simulink model "ISReferenceApplication"  (R2018a)
settings: Solver=FixedStepAuto  StartTime=0  StopTime=Tend  FixedStep=0.001  RelTol=5e-3
model workspace (MAT data in the model file):
  A_mu = 10
  B_reff = 8.386
  Cz = 7766.25
  DCT_Param.Transmission.Ratios = [3.78 2.18 1.43 1.03 0.935 0.84]
  DCT_Param.Transmission.Shaft_Inertia_Odd = 0.0023
  DCT_Param.Transmission.Shaft_Inertia_Even = 0.0009
  DCT_Param.Transmission.Shaft_Inertia_Output = 0.008
  DCT_Param.Transmission.Gear_Inertia = 0.001
  DCT_Param.Transmission.Gear_Efficiency = 0.94
  DCT_Param.Transmission.Gear_Ang_Vel_Thr = 0.01
  DCT_Param.Transmission.Shaft_Velocity_Odd = 0
  DCT_Param.Transmission.Shaft_Velocity_Even = 0
  DCT_Param.Transmission.Shaft_Velocity_Output = 0
  DCT_Param.Transmission.Gear_Initial_Velocity = 0
  DCT_Param.Transmission.Abstract.Compliance = 100000
  DCT_Param.Transmission.Abstract.Damping = 10000
  DCT_Param.Transmission.Abstract.Ratio_Time_Const = 0.05
  DCT_Param.Transmission.Abstract.Shift_Gear_Delay = 25
  DCT_Param.Clutch.Torque_Radius = 130
  DCT_Param.Clutch.Num_Friction_Surfaces = 4
  DCT_Param.Clutch.Engagement_Piston_Area = 0.001
  DCT_Param.Clutch.Kinetic_Friction_Coeff = 0.3
  DCT_Param.Clutch.Static_Friction_Coeff = 0.31
  DCT_Param.Clutch.Derating_Factor = 1
  DCT_Param.Clutch.Clutch_Velocity_Tolerance = 0.001
  DCT_Param.Clutch.Threshold_Pressure = 1
  DCT_Param.Clutch.Drag_Torque_Coeff = 0
  DCT_Param.Dog_Clutch.Max_Torque = 1000
  DCT_Param.Dog_Clutch.Teeth_Mean_Radius = 50
  DCT_Param.Dog_Clutch.Tooth_Height = 10
  DCT_Param.Dog_Clutch.Ring_Hub_Clearance = 3
  DCT_Param.Dog_Clutch.Ring_Stop_Stiffness = 1000000
  DCT_Param.Dog_Clutch.Ring_Stop_Damping = 1000
  DCT_Param.Dog_Clutch.Shift_Linkage_Damping = 100
  DCT_Param.Dog_Clutch.Max_Engage_Velocity = 1000000
  DCT_Param.Dog_Clutch.Tooth_Engage_Overlap = 3
  DCT_Param.Vehicle.Mass = 1600
  DCT_Param.Vehicle.Wheels_Per_Axle = 2
  DCT_Param.Vehicle.Distance_CG_FrontAxle = 1.7
  DCT_Param.Vehicle.Distance_CG_RearAxle = 2
  DCT_Param.Vehicle.Distance_CG_Ground = 0.5
  DCT_Param.Vehicle.Frontal_Area = 3
  DCT_Param.Vehicle.Aero_Drag_Coeff = 0.4
  DCT_Param.Vehicle.Initial_Velocity = 0
  DCT_Param.Vehicle.Final_Drive_Ratio = 3.7
  DCT_Param.Vehicle.Final_Drive_Efficiency = 0.86
  DCT_Param.Vehicle.Final_Drive_Vel_Thresh = 0.01
  DCT_Param.Vehicle.Side_Shaft_Inertia = 0.01
  DCT_Param.Vehicle.Side_Shaft_Initial_Velocity = 0
  DCT_Param.Vehicle.Tire.Radius = 0.312
  DCT_Param.Vehicle.Tire.Inertia = 0.5
  DCT_Param.Vehicle.Tire.Initial_Velocity = 0
  DCT_Param.Vehicle.Tire.Slip_Vel_Thresh = 0.1
  DCT_Param.Vehicle.Tire.Nominal_Vertical_Load = 4000
  DCT_Param.Vehicle.Tire.C_Coeff = 1.685
  DCT_Param.Vehicle.Tire.D_Coeff = [1.21 -0.037]
  DCT_Param.Vehicle.Tire.E_Coeff = [0.344 0.095 -0.02 0]
  DCT_Param.Vehicle.Tire.BCD_Coeff = [21.51 -0.163 0.245]
  DCT_Param.Vehicle.Tire.H_Coeff = [-0.002 0.002]
  DCT_Param.Vehicle.Tire.V_Coeff = [0 0]
  DCT_Param.ICE.Max_Power = 100000
  DCT_Param.ICE.Speed_At_Max_Power = 5500
  DCT_Param.ICE.Max_Speed = 7000
  DCT_Param.ICE.Stall_Speed = 200
  DCT_Param.ICE.Shaft_Inertia = 0.2
  DCT_Param.ICE.Initial_Velocity = 800
  DCT_Param.ICE.Idle_Ref_Spd = 800
  DCT_Param.ICE.Engine_Time_Constant = 0.2
  DCT_Param.ICE.Initial_Normalized_Throttle = 0
  DCT_Param.ICE.Speed_Threshold = 20
  DCT_Param.ICE.FC.Speed_Vector = [0 368.421052632 736.842105263 1105.26315789 1473.68421053 1842.10526316 2210.52631579 2578.94736842 2947.36842105 3315.78947368 3684.21052632 4052.63157895 4421.05263158 4789.47368421 5157.89473684 5526.31578947 5894.73684211 6263.15789474 6631.57894737 7000]
  DCT_Param.ICE.FC.Torque_Vector = [0 10.5263157895 21.0526315789 31.5789473684 42.1052631579 52.6315789474 63.1578947368 73.6842105263 84.2105263158 94.7368421053 105.263157895 115.789473684 126.315789474 136.842105263 147.368421053 157.894736842 168.421052632 178.947368421 189.473684211 200]
  DCT_Param.ICE.FC.Consumption_Table = [0.262945178015 0.225304787522 0.201465019624 0.191425874321 0.195187351614 0.212749451502 0.244112173984 0.289275519063 0.348239486736 0.421004077004 0.507569289868 0.607935125326 ... (400 elements, 20x20)]
  DCT_Param.Shift_Map_Example.Pedal_Positions = [0.1 0.4 0.5 0.9]
  DCT_Param.Shift_Map_Example.Upshift_Speeds = [11  20  26  34.5  43; 14  26  35  44.5  55; 17  31  42  52.5  65; 21  39  52  66.5  80]
  DCT_Param.Shift_Map_Example.Downshift_Speeds = [8.9  17  23.6  32.4  40.8; 11.5  22.7  32  41.6  52.2; 14  27  38.1  50  62; 18  33  48  62.6  76.2]
  DCT_Param.Shift_Map_ORIG.Pedal_Positions = [0.1 0.4 0.5 0.9]
  DCT_Param.Shift_Map_ORIG.Upshift_Speeds = [11.5  23.5  35.5  45.5  55.5; 14.5  26.5  38.5  48.5  58.5; 17.5  29.5  41.5  51.5  61.5; 20.5  32.5  44.5  54.5  64.5]
  DCT_Param.Shift_Map_ORIG.Downshift_Speeds = [8.5  20.5  32.5  42.5  52.5; 11.5  23.5  35.5  45.5  55.5; 14.5  26.5  38.5  48.5  58.5; 17.5  29.5  41.5  51.5  61.5]
  DCT_Param.Shift_Map_OPT.Pedal_Positions = [0.1 0.4 0.5 0.9]
  DCT_Param.Shift_Map_OPT.Upshift_Speeds = [17.8469  29.8469  35.8159  41.2981  46.3004; 19.2469  33.9778  43.9778  53.9778  63.9778; 24.5469  41.9778  62.1778  78.5778  106.9778; 27.5469  59.3778  99.0445  109.0445  119.0445]
  DCT_Param.Shift_Map_OPT.Downshift_Speeds = [14.8469  26.8469  32.8159  38.2981  43.3004; 16.2469  30.9778  40.9778  50.9778  60.9778; 21.5469  38.9778  59.1778  75.5778  103.9778; 24.5469  56.3778  96.0445  106.0445  116.0445]
  DCT_Param.Shift_Map.Pedal_Positions = [0.1 0.4 0.5 0.9]
  DCT_Param.Shift_Map.Upshift_Speeds = [11.5  23.5  35.5  45.5  55.5; 14.5  26.5  38.5  48.5  58.5; 17.5  29.5  41.5  51.5  61.5; 20.5  32.5  44.5  54.5  64.5]
  DCT_Param.Shift_Map.Downshift_Speeds = [8.5  20.5  32.5  42.5  52.5; 11.5  23.5  35.5  45.5  55.5; 14.5  26.5  38.5  48.5  58.5; 17.5  29.5  41.5  51.5  61.5]
  DCT_Param.Control.Clutch.Min_Lock_Pressure = 2000000
  DCT_Param.Control.Clutch.Max_Lock_Pressure = 5000000
  DCT_Param.Control.Clutch.Max_Unlock_Pressure = 500000
  DCT_Param.Control.Engine_Start_RPM = 800
  DCT_Param.Control.Engine_Stop_RPM = 790
  DCT_Param.Control.Mode_Logic_TS = 0.1
  DCT_Param.Control.ICE.Kp = 0.02
  DCT_Param.Control.ICE.Ki = 0.01
  DCT_Param.Control.Gen.Kp = 10
  DCT_Param.Control.Gen.Ki = 3
  DCT_Param.Control.Mot.Kp = 500
  DCT_Param.Control.Mot.Ki = 300
  DCT_Param.Control.Veh_Spd.Kp = 0.02
  DCT_Param.Control.Veh_Spd.Ki = 0.04
  DCT_Param.Driver.Kp = 400
  DCT_Param.Driver.Ki = 0.001
  DCT_Param.Driver.Pedal_Filter_Const = 0.01
  DCT_Param.Dog_Clutches.Pulse_Delay = 50
  DCT_Param.Dog_Clutches.Pulse_Length = 20
  DCT_Param.Animation.Teeth_Ratios = [0.338461538462 0.555555555556 0.916666666667 0.96 1.17948717949 1.92307692308]
  DCT_Param.Animation.Teeth_Ratios_Reverse = [0.458333333333 0.75]
  DCT_Param.Shift_Map_OPT506.Pedal_Positions = [0.1 0.4 0.5 0.9]
  DCT_Param.Shift_Map_OPT506.Upshift_Speeds = [18  30.2  48.3  67.3322  77.3429; 20.1  36.85  66.6178  76.7537  86.7537; 21.1  40.25  71.0189  81.0189  91.7873; 24.1  63.75  80.7523  105.9489  115.9489]
  DCT_Param.Shift_Map_OPT506.Downshift_Speeds = [15  27.2  45.3  64.3322  74.3429; 17.1  33.85  63.6178  73.7537  83.7537; 18.1  37.25  68.0189  78.0189  88.7873; 21.1  60.75  77.7523  102.9489  112.9489]
  DCT_Param.Shift_Map_OPTAbsRea176.Pedal_Positions = [0.1 0.4 0.5 0.9]
  DCT_Param.Shift_Map_OPTAbsRea176.Upshift_Speeds = [17.8469  29.8469  35.7875  44.0901  49.4243; 18.9219  34.1312  45.8256  59.7585  69.7585; 32.1719  43.4585  53.51  103.2151  114.6401; 35.1719  59.2585  99.5217  109.5217  119.5217]
  DCT_Param.Shift_Map_OPTAbsRea176.Downshift_Speeds = [14.8469  26.8469  32.7875  41.0901  46.4243; 15.9219  31.1312  42.8256  56.7585  66.7585; 29.1719  40.4585  50.51  100.2151  111.6401; 32.1719  56.2585  96.5217  106.5217  116.5217]
  D_reff = 0.25826
  Downshift_Speeds = [9.5625  23.0625  36.5625  47.8125  59.0625  68.90625  78.75; 12.9375  26.4375  39.9375  51.1875  62.4375  72.84375  83.25; 16.3125  29.8125  43.3125  54.5625  65.8125  76.78125  87.75; 19.6875  33.1875  46.6875  57.9375  69.1875  80.71875  92.25]
  Pedal_Positions = [0.1 0.4 0.5 0.9]
  SUS.Stiffness = 24000
  SUS.Damping.Constant = 1262
  SUS.Damping.Rebound = [4040 4950 2883 2043]
  SUS.Damping.Compression = [3600 3420 1863 1472]
  SUS.PistonSpeed = [0.05 0.1 0.3 0.6]
  SUS.UnsprungMass.Fr = 21.0693333333
  SUS.UnsprungMass.Rr = 21.0693333333
  Upshift_Speeds = [12.9375  26.4375  39.9375  51.1875  62.4375  72.84375  83.25; 16.3125  29.8125  43.3125  54.5625  65.8125  76.78125  87.75; 19.6875  33.1875  46.6875  57.9375  69.1875  80.71875  92.25; 33  52.5  77.25  100.5  138.75  161.875  185]
  VEH.Mass = 1181
  VEH.StaticNormalFrontLoad.FR = 264.666666667
  VEH.StaticNormalFrontLoad.FL = 264.666666667
  VEH.StaticNormalRearLoad.RR = 322
  VEH.StaticNormalRearLoad.RL = 322
  VEH.WheelBase = 3.075
  VEH.FrontAxlePositionfromCG = 1.515
  VEH.RearAxlePositionfromCG = 1.504
  VEH.HeightCG = 0.134
  VEH.FrontalArea = 2.11
  VEH.DragCoefficient = 0.33
  VEH.NumberOfWheelsPerAxle = 2
  VEH.Thread.FR = 1.705
  VEH.Thread.RR = 1.705
  VEH.PitchMomentInertia = 1922.66666667
  VEH.RollMomentInertia = 432.333333333
  VEH.YawMomentInertia = 2066
  VEH.SteeringRatio = 18
  VEH.TrackWidth = 1.922
  VEH.SprungMass = 1096.72266667
  VEH.InitialLongPosition = 0
  VEH.InitialLatPosition = 3.125
  VEH.InitialVertPosition = 0.0111
  VEH.InitialRollAngle = 0
  VEH.InitialPitchAngle = -0.000732
  VEH.InitialYawAngle = 0
  VEH.InitialLongVel = 0
  VEH.InitialLatVel = 0
  VEH.InitialVertVel = 0
  VEH.InitialRollRate = 0
  VEH.InitialPitchRate = 0
  VEH.InitialYawRate = 0
  V_o = 16.7
  V_xlow = 1
  WH.Tire.Radius.Front = 0.384
  WH.Tire.Radius.Rear = 0.401
  WH.Tire.Sidewall = 0.245
  WH.Tire.RollingResistCoeff = 0.0103
  WH.Tire.Magic.B = 10
  WH.Tire.Magic.C = 1.9
  WH.Tire.Magic.D = 1
  WH.Tire.Magic.E = 0.97
  WH.Tire.Magic.Bx = 12
  WH.Tire.Magic.Cx = 1.9
  WH.Tire.Magic.Dx = 0.72
  WH.Tire.Magic.Ex = 0.95
  WH.Tire.Magic.By = 12
  WH.Tire.Magic.Cy = 1.3
  WH.Tire.Magic.Dy = 0.75
  WH.Tire.Magic.Ey = 0.2
  WH.Tire.Front.Ky = 40000
  WH.Tire.Rear.Ky = 40000
  WH.Tire.Kz = 320000
  WH.Tire.Damping = 100
  WH.Inertia = 1.00333333333
  WH.Mass = 11.4333333333
  WH.DampingCoefficient = 0.01
  WH.VelocityTol = 0.1
  a = 1.4
  alpha_max = 1.5
  alpha_min = -1.5
  b = 1.8
  c_zo = 209651
  epsilon = 0.1
  h = 0.134
  path.ISO3888p2.x = [0 2 12 25.5 36.5 49 61]
  path.ISO3888p2.y = [0 0 0 3.725 3.725 0 0]
  path.ISO3888p2.ylb = [1.225 1.225 1.225 4.725 4.725 1.5 1.5]
  path.ISO3888p2.yrb = [-1.225 -1.225 -1.225 2.225 2.225 -1.5 -1.5]
  path.CUSC.x = [10.668 21.336 36.576 54.864 73.152]
  path.CUSC.y = [0 0 5.1816 0 0]
  path.CUSC.ylb = [1.2192 1.2192 7.0104 1.8288 1.8288]
  path.CUSC.yrb = [-1.2192 -1.2192 3.3528 -1.8288 -1.8288]
  pio = 220000
  q_Fcx = 0
  q_Fz2 = 15.4
  q_Fzy = 0
  q_reo = 0.9974
  q_sx1 = -0.007764
  q_sx10 = 0.2824
  q_sx11 = 5.349
  q_sx12 = 0
  q_sx13 = 0
  q_sx14 = 0
  q_sx2 = 1.1915
  q_sx3 = 0.013948
  q_sx4 = 4.912
  q_sx5 = 1.02
  q_sx6 = 22.83
  q_sx7 = 0.7104
  q_sx8 = -0.023393
  q_sx9 = 0.6581
  q_sy1 = 0.00702
  q_sy2 = 0
  q_sy3 = 0.001515
  q_sy4 = 8.514e-05
  q_sy5 = 0
  q_sy6 = 0
  q_sy7 = 0.9008
  q_sy8 = -0.4089
  q_v1 = 0.0007742
  q_v2 = 0.04667
  r_Bx1 = 12.531
  r_Bx2 = 9.532
  r_Bx3 = 0
  r_By1 = 10.615
  r_By2 = 7.705
  r_By3 = 3.433e-06
  r_By4 = 0
  r_Cx1 = 1.019
  r_Cy1 = 1.0585
  r_Ex1 = -0.4487
  r_Ex2 = -0.4726
  r_Ey1 = 0.3132
  r_Ey2 = 7.63e-06
  r_Hx1 = 0.0002374
  r_Hy1 = 0.011646
  r_Hy2 = 7.63e-06
  r_Vy1 = 0.05654
  r_Vy2 = 7.63e-06
  r_Vy3 = 0
  r_Vy4 = 99.9
  r_Vy5 = 2
  r_Vy6 = 15.814
  r_o = 0.3135
  vehWidth = 2
  w = 1
undefined symbols (not defined in the file): Cok_1, Cok_2, Cok_3, Cok_4, Cok_5, Cok_6, Cok_7, Cok_8, Cok_9, Cout_1, Cout_2, Cout_3, Cout_4, Cout_5, Cout_6, Cout_7, Cout_8, Cout_9, Dout_1, Dout_2, Dout_3, Dout_4, Dout_5, Dout_6, Dout_7, Dout_8, Dout_9, F_1, F_2, F_3, F_4, F_5, F_6, F_7, F_8, F_9, Gd_1, Gd_2, Gd_3, Gd_4, Gd_5, Gd_6, Gd_7, Gd_8, Gd_9, Gok_1, Gok_2, Gok_3, Gok_4, Gok_5, Gok_6, Gok_7, Gok_8, Gok_9, Hd_1, Hd_2, Hd_3, Hd_4, Hd_5, Hd_6 ... (+64)
(part 1 of 3)
settings Model: ModifiedByFormat=The MathWorks, Inc.  Creator=The MathWorks, Inc.  LastModifiedBy=The MathWorks, Inc.
settings SolverCC: ZeroCrossAlgorithm=Adaptive  AlgebraicLoopSolver=LineSearch  DecoupledContinuousIntegration=on  MinimalZcImpactIntegration=on
settings DebuggingCC: SignalInfNanChecking=error  ArtificialAlgebraicLoopMsg=none  IgnoredZcDiagnostic=none  ModelReferenceExtraNoncontSigs=none
settings ModelReferenceCC: UpdateModelReferenceTargets=IfOutOfDate  EnableParallelModelReferenceBuilds=on  ModelReferenceMinAlgLoopOccurrences=on  PropagateSignalLabelsOutOfModel=off
settings RTWCC: BuildConfiguration=Faster Runs

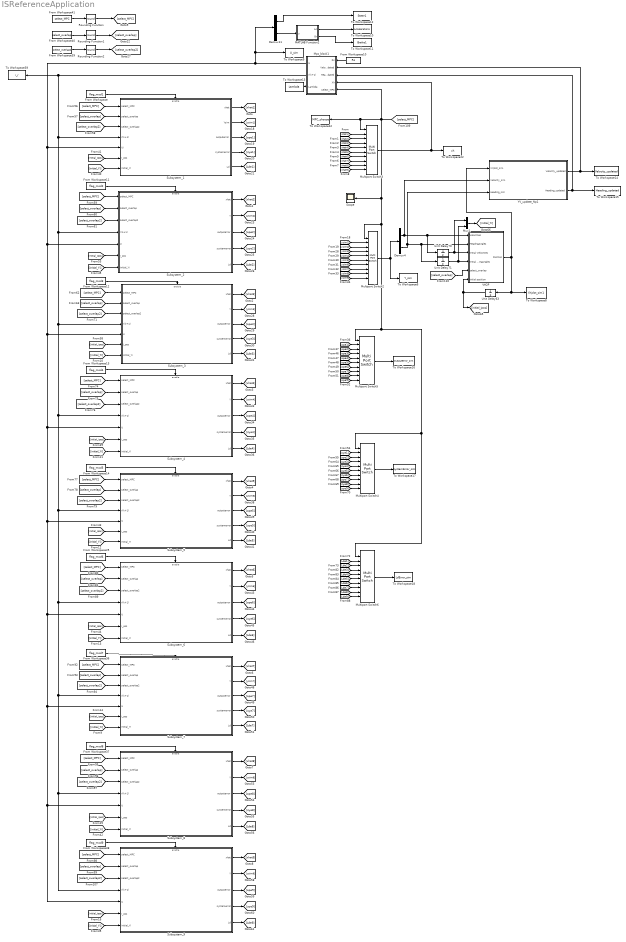
== system ISReferenceApplication ==
  Demux11 : Demux  Outputs=2
  Demux4 : Demux  Outputs=2
  From Workspace : FromWorkspace  VariableName=flag_mod1  SampleTime=0
  From Workspace10 : FromWorkspace  VariableName=Rs  SampleTime=Ts
  From Workspace11 : FromWorkspace  VariableName=flag_mod2  SampleTime=0
  From Workspace12 : FromWorkspace  VariableName=flag_mod3  SampleTime=0
  From Workspace13 : FromWorkspace  VariableName=flag_mod4  SampleTime=0
  From Workspace14 : FromWorkspace  VariableName=flag_mod5  SampleTime=0
  From Workspace25 : FromWorkspace  VariableName=flag_mod6  SampleTime=0
  From Workspace36 : FromWorkspace  VariableName=flag_mod7  SampleTime=0
  From Workspace37 : FromWorkspace  VariableName=flag_mod8  SampleTime=0
  From Workspace38 : FromWorkspace  VariableName=flag_mod9  SampleTime=0
  From Workspace39 : FromWorkspace  VariableName=select_overlap2  SampleTime=Ts
  From Workspace40 : FromWorkspace  VariableName=select_overlap  SampleTime=Ts
  From Workspace41 : FromWorkspace  VariableName=select_MPC  SampleTime=Ts
  MATLAB Function2 : MATLAB Function  TreatAsAtomicUnit=on  SystemSampleTime=Ts
  Mpc_block1 : Subsystem  TreatAsAtomicUnit=on  SystemSampleTime=Ts
  Multiport Switch{2..6} (5 alike) : MultiPortSwitch  Inputs=9
  Mux1 : Mux  Inputs=2
  Rounding Function : Rounding  Operator=round
  Rounding Function1 : Rounding  Operator=round
  Rounding Function2 : Rounding  Operator=round
  Scope : Scope
  Subsystem_1 : Subsystem
  Subsystem_2 : Subsystem
  Subsystem_3 : Subsystem
  Subsystem_4 : Subsystem
  Subsystem_5 : Subsystem
  Subsystem_6 : Subsystem
  Subsystem_7 : Subsystem
  Subsystem_8 : Subsystem
  Subsystem_9 : Subsystem
  To Workspace10 : ToWorkspace  VariableName=Acceleration1  SampleTime=Ts
  To Workspace11 : ToWorkspace  VariableName=Brake1  SampleTime=Ts
  To Workspace12 : ToWorkspace  VariableName=Steer1  SampleTime=Ts
  To Workspace13 : ToWorkspace  VariableName=Lambda  SampleTime=Ts
  To Workspace14 : ToWorkspace  VariableName=Velocity_updated  SampleTime=Ts
  To Workspace15 : ToWorkspace  VariableName=Heading_updated  SampleTime=Ts
  To Workspace16 : ToWorkspace  VariableName=OutputError_sim  SampleTime=Ts
  To Workspace17 : ToWorkspace  VariableName=SystemError_sim  SampleTime=Ts
  To Workspace18 : ToWorkspace  VariableName=LdError_sim  SampleTime=Ts
  To Workspace22 : ToWorkspace  VariableName=xh  SampleTime=-1
  To Workspace39 : ToWorkspace  VariableName=i_r  SampleTime=Ts
  To Workspace42 : ToWorkspace  VariableName=MPC_choose  SampleTime=-1
  To Workspace6 : ToWorkspace  VariableName=Y_sim  SampleTime=Ts
  To Workspace8 : ToWorkspace  VariableName=XYplot_sim1  SampleTime=Ts
  To Workspace9 : ToWorkspace  VariableName=U_sim  SampleTime=Ts
  Unit Delay63 : UnitDelay  SampleTime=Ts
  Unit Delay70 : UnitDelay  InitialCondition=ro(1,:)  SampleTime=Ts
  Unit Delay71 : UnitDelay  InitialCondition=ro(2,:)  SampleTime=Ts
  VH2P : Subsystem
  YV_update_Np1 : Subsystem  TreatAsAtomicUnit=on
  wires:
  From Workspace10/1 -> Mpc_block1/1(Rs)
  Unit Delay63/1 -> [initial_ipos], VH2P/6(Initial position)
  Demux4/2 -> Unit Delay71/1, VH2P/2(HeadingAngles), YV_update_Np1/3(Heading_sim)
  YV_update_Np1/1(Velocity_updated) -> Mpc_block1/2(Velocity_updated), To Workspace14/1
  Multiport Switch3/1 -> Mpc_block1/4(Xh), To Workspace22/1
  [select_overlap] -> Subsystem_1/2(select_overlap)
  [select_overlap] -> Subsystem_3/2(select_overlap)
  Demux11/2 -> MATLAB Function2/1(u)
  MATLAB Function2/1(Ac) -> To Workspace10/1
  MATLAB Function2/2(Br) -> To Workspace11/1
  Demux11/1 -> To Workspace12/1
  Mpc_block1/3(Lambda) -> To Workspace13/1
  YV_update_Np1/2(Heading_updated) -> Mpc_block1/3(Heading_updated), To Workspace15/1
  VH2P/1(Position) -> To Workspace8/1, Unit Delay63/1, YV_update_Np1/1(XYplot_sim)
  [select_overlap] -> Subsystem_9/2(select_overlap)
  Multiport Switch5/1 -> To Workspace16/1
  Multiport Switch4/1 -> To Workspace17/1
  Multiport Switch6/1 -> To Workspace18/1
  [select_overlap] -> VH2P/5(select_overlap)
  Unit Delay70/1 -> Mux1/1, VH2P/3(Iintial Velocities)
  Unit Delay71/1 -> Mux1/2, VH2P/4(Iintial HeadingAngles)
  Demux4/1 -> VH2P/1(Velocities), Unit Delay70/1, YV_update_Np1/2(Velocity_sim)
  [select_MPC] -> Subsystem_1/1(select_MPC)
  [select_overlap] -> Subsystem_2/2(select_overlap)
  [select_overlap] -> Subsystem_4/2(select_overlap)
  [select_overlap] -> Subsystem_5/2(select_overlap)
  [select_overlap] -> Subsystem_6/2(select_overlap)
  [select_overlap] -> Subsystem_7/2(select_overlap)
  [select_overlap] -> Subsystem_8/2(select_overlap)
  [select_MPC] -> Subsystem_2/1(select_MPC)
  [select_MPC] -> Subsystem_3/1(select_MPC)
  [select_MPC] -> Subsystem_4/1(select_MPC)
  [select_MPC] -> Subsystem_5/1(select_MPC)
  [select_MPC] -> Subsystem_6/1(select_MPC)
  [select_MPC] -> Subsystem_7/1(select_MPC)
  [select_MPC] -> Subsystem_8/1(select_MPC)
  [select_MPC] -> Subsystem_9/1(select_MPC)
  [select_overlap2] -> Subsystem_1/3(select_overlap2)
  [select_overlap2] -> Subsystem_2/3(select_overlap2)
  [select_overlap2] -> Subsystem_3/3(select_overlap2)
  [select_overlap2] -> Subsystem_4/3(select_overlap2)
  [select_overlap2] -> Subsystem_5/3(select_overlap2)
  [select_overlap2] -> Subsystem_6/3(select_overlap2)
  [select_overlap2] -> Subsystem_7/3(select_overlap2)
  [select_overlap2] -> Subsystem_8/3(select_overlap2)
  [select_overlap2] -> Subsystem_9/3(select_overlap2)
  Mpc_block1/1(U) -> Demux11/1, To Workspace9/1, Subsystem_9/5(U), Subsystem_8/5(U), Subsystem_7/5(U), Subsystem_6/5(U), Subsystem_5/5(U), Subsystem_4/5(U), Subsystem_3/5(U), Subsystem_2/5(U), Subsystem_1/5(Ui)
  Mpc_block1/2(r(k+1)) -> Subsystem_9/4(r(k+1)), Subsystem_8/4(r(k+1)), Subsystem_7/4(r(k+1)), Subsystem_6/4(r(k+1)), Subsystem_5/4(r(k+1)), Subsystem_4/4(r(k+1)), Subsystem_3/4(r(k+1)), Subsystem_2/4(r(k+1)), Subsystem_1/4(r(k+1)), To Workspace39/1
  Subsystem_1/1(xhat) -> [xhat1]
  [xhat1] -> Multiport Switch3/2
  [xhat2] -> Multiport Switch3/3
  [xhat8] -> Multiport Switch3/9
  [xhat3] -> Multiport Switch3/4
  [xhat4] -> Multiport Switch3/5
  [xhat5] -> Multiport Switch3/6
  [xhat6] -> Multiport Switch3/7
  [xhat7] -> Multiport Switch3/8
  [xhat9] -> Multiport Switch3/10
  Subsystem_3/1(xhat) -> [xhat3]
  Subsystem_4/1(xhat) -> [xhat4]
  Subsystem_5/1(xhat) -> [xhat5]
  Subsystem_7/1(xhat) -> [xhat7]
  Subsystem_8/1(xhat) -> [xhat8]
  Subsystem_9/1(xhat) -> [xhat9]
  [ysim8] -> Multiport Switch2/9
  [ysim1] -> Multiport Switch2/2
  [ysim2] -> Multiport Switch2/3
  [ysim5] -> Multiport Switch2/6
  [ysim6] -> Multiport Switch2/7
  [ysim7] -> Multiport Switch2/8
  [ysim4] -> Multiport Switch2/5
  [ysim9] -> Multiport Switch2/10
  [ysim3] -> Multiport Switch2/4
  [ope8] -> Multiport Switch5/9
  [ope1] -> Multiport Switch5/2
  [ope2] -> Multiport Switch5/3
  [ope5] -> Multiport Switch5/6
  [ope6] -> Multiport Switch5/7
  [ope7] -> Multiport Switch5/8
  [ope4] -> Multiport Switch5/5
  [ope9] -> Multiport Switch5/10
  [ope3] -> Multiport Switch5/4
  [sye8] -> Multiport Switch4/9
  [sye1] -> Multiport Switch4/2
  [sye2] -> Multiport Switch4/3
  [sye5] -> Multiport Switch4/6
  [sye6] -> Multiport Switch4/7
  [sye7] -> Multiport Switch4/8
  [sye4] -> Multiport Switch4/5
  [sye9] -> Multiport Switch4/10
  [sye3] -> Multiport Switch4/4
  [Lde8] -> Multiport Switch6/9
  [Lde1] -> Multiport Switch6/2
  [Lde2] -> Multiport Switch6/3
  [Lde5] -> Multiport Switch6/6
  [Lde6] -> Multiport Switch6/7
  [Lde7] -> Multiport Switch6/8
  [Lde4] -> Multiport Switch6/5
  [Lde9] -> Multiport Switch6/10
  [Lde3] -> Multiport Switch6/4
  Subsystem_1/2(Ysim) -> [ysim1]
  Subsystem_1/3(outputerror) -> [ope1]
  Subsystem_1/4(systemerror) -> [sye1]
  Subsystem_1/5(Ld) -> [Lde1]
  Subsystem_2/2(Y) -> [ysim2]
  Subsystem_2/3(outputerror) -> [ope2]
  Subsystem_2/4(systemerror) -> [sye2]
  Subsystem_2/5(Ld) -> [Lde2]
  Subsystem_3/2(Y) -> [ysim3]
  Subsystem_3/3(outputerror) -> [ope3]
  Subsystem_3/4(systemerror) -> [sye3]
  Subsystem_3/5(Ld) -> [Lde3]
  Subsystem_4/2(Y) -> [ysim4]
  Subsystem_4/3(outputerror) -> [ope4]
  Subsystem_4/4(systemerror) -> [sye4]
  Subsystem_4/5(Ld) -> [Lde4]
  Subsystem_5/2(Y) -> [ysim5]
  Subsystem_5/3(outputerror) -> [ope5]
  Subsystem_5/4(systemerror) -> [sye5]
  Subsystem_5/5(Ld) -> [Lde5]
  Subsystem_6/3(outputerror) -> [ope6]
  Subsystem_6/4(systemerror) -> [sye6]
  Subsystem_6/5(Ld) -> [Lde6]
  Subsystem_7/2(Y) -> [ysim7]
  Subsystem_7/3(outputerror) -> [ope7]
  Subsystem_7/4(systemerror) -> [sye7]
  Subsystem_7/5(Ld) -> [Lde7]
  Subsystem_8/2(Y) -> [ysim8]
  Subsystem_8/3(outputerror) -> [ope8]
  Subsystem_8/4(systemerror) -> [sye8]
  Subsystem_8/5(Ld) -> [Lde8]
  Subsystem_9/2(Y) -> [ysim9]
  Subsystem_9/3(outputerror) -> [ope9]
  Subsystem_9/4(systemerror) -> [sye9]
  Subsystem_9/5(Ld) -> [Lde9]
  Subsystem_2/1(xhat) -> [xhat2]
  From Workspace38/1 -> Subsystem_9/Enable
  From Workspace11/1 -> Subsystem_2/Enable
  Multiport Switch2/1 -> To Workspace6/1, Demux4/1
  Subsystem_6/1(xhat) -> [xhat6]
  Subsystem_6/2(Y) -> [ysim6]
  [select_MPC] -> To Workspace42/1, Multiport Switch3/1, Mpc_block1/5(select_MPC), Scope/1, Multiport Switch2/1, Multiport Switch6/1, Multiport Switch4/1, Multiport Switch5/1
  From Workspace/1 -> Subsystem_1/Enable
  From Workspace13/1 -> Subsystem_4/Enable
  From Workspace36/1 -> Subsystem_7/Enable
  From Workspace12/1 -> Subsystem_3/Enable
  From Workspace14/1 -> Subsystem_5/Enable
  From Workspace25/1 -> Subsystem_6/Enable
  From Workspace37/1 -> Subsystem_8/Enable
  Mux1/1 -> [initial_Yi]
  [initial_ipos] -> Subsystem_1/6(i_pos)
  [initial_Yi] -> Subsystem_1/7(initial_Yi)
  [initial_Yi] -> Subsystem_4/7(initial_Yi)
  [initial_ipos] -> Subsystem_4/6(i_pos)
  [initial_ipos] -> Subsystem_7/6(i_pos)
  [initial_Yi] -> Subsystem_7/7(initial_Yi)
  [initial_Yi] -> Subsystem_3/7(initial_Yi)
  [initial_ipos] -> Subsystem_3/6(i_pos)
  [initial_ipos] -> Subsystem_8/6(i_pos)
  [initial_Yi] -> Subsystem_8/7(initial_Yi)
  [initial_ipos] -> Subsystem_5/6(i_pos)
  [initial_Yi] -> Subsystem_5/7(initial_Yi)
  [initial_ipos] -> Subsystem_6/6(i_pos)
  [initial_Yi] -> Subsystem_6/7(initial_Yi)
  [initial_Yi] -> Subsystem_2/7(initial_Yi)
  [initial_ipos] -> Subsystem_2/6(i_pos)
  [initial_ipos] -> Subsystem_9/6(i_pos)
  [initial_Yi] -> Subsystem_9/7(initial_Yi)
  From Workspace39/1 -> Rounding Function2/1
  Rounding Function2/1 -> [select_overlap2]
  From Workspace40/1 -> Rounding Function1/1
  Rounding Function1/1 -> [select_overlap]
  From Workspace41/1 -> Rounding Function/1
  Rounding Function/1 -> [select_MPC]

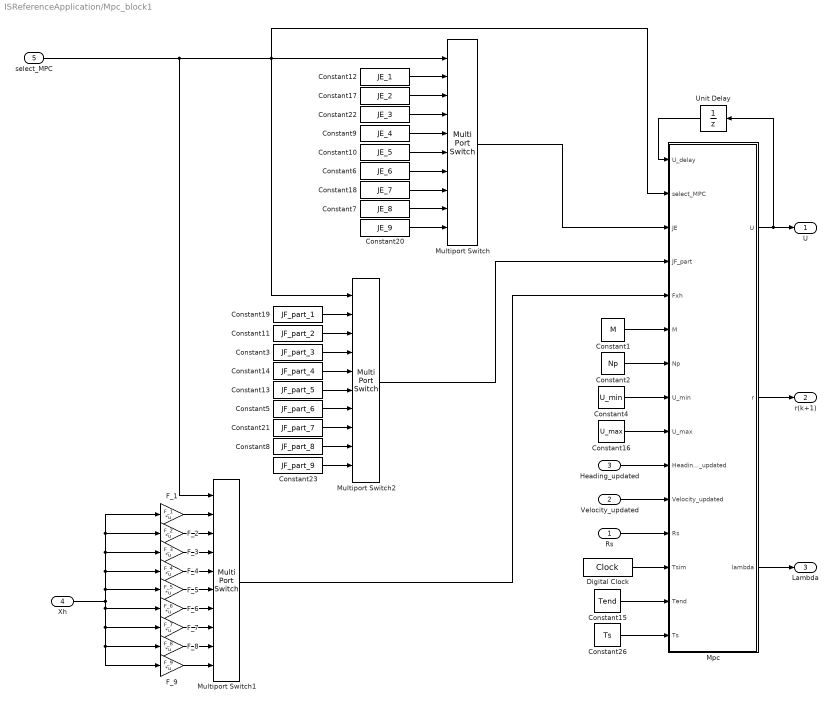
== system ISReferenceApplication/Mpc_block1 ==
  Rs : Inport  SampleTime=Ts  LockScale=on
  Velocity_updated : Inport  Port=2  SampleTime=Ts
  Heading_updated : Inport  Port=3  SampleTime=Ts  LockScale=on
  Xh : Inport  Port=4
  select_MPC : Inport  Port=5
  Constant1 : Constant  Value=M  VectorParams1D=off  SampleTime=-1
  Constant10 : Constant  Value=JE_5  VectorParams1D=off  SampleTime=-1
  Constant11 : Constant  Value=JF_part_2  VectorParams1D=off  SampleTime=-1
  Constant12 : Constant  Value=JE_1  VectorParams1D=off  SampleTime=-1
  Constant13 : Constant  Value=JF_part_5  VectorParams1D=off  SampleTime=-1
  Constant14 : Constant  Value=JF_part_4  VectorParams1D=off  SampleTime=-1
  Constant15 : Constant  Value=Tend  VectorParams1D=off  SampleTime=-1
  Constant16 : Constant  Value=U_max  VectorParams1D=off  SampleTime=-1
  Constant17 : Constant  Value=JE_2  VectorParams1D=off  SampleTime=-1
  Constant18 : Constant  Value=JE_7  VectorParams1D=off  SampleTime=-1
  Constant19 : Constant  Value=JF_part_1  VectorParams1D=off  SampleTime=-1
  Constant2 : Constant  Value=Np  SampleTime=-1
  Constant20 : Constant  Value=JE_9  VectorParams1D=off  SampleTime=-1
  Constant21 : Constant  Value=JF_part_7  VectorParams1D=off  SampleTime=-1
  Constant22 : Constant  Value=JE_3  VectorParams1D=off  SampleTime=-1
  Constant23 : Constant  Value=JF_part_9  VectorParams1D=off  SampleTime=-1
  Constant26 : Constant  Value=Ts  VectorParams1D=off  SampleTime=-1
  Constant3 : Constant  Value=JF_part_3  VectorParams1D=off  SampleTime=-1
  Constant4 : Constant  Value=U_min  VectorParams1D=off  SampleTime=-1
  Constant5 : Constant  Value=JF_part_6  VectorParams1D=off  SampleTime=-1
  Constant6 : Constant  Value=JE_6  VectorParams1D=off  SampleTime=-1
  Constant7 : Constant  Value=JE_8  VectorParams1D=off  SampleTime=-1
  Constant8 : Constant  Value=JF_part_8  VectorParams1D=off  SampleTime=-1
  Constant9 : Constant  Value=JE_4  VectorParams1D=off  SampleTime=-1
  Digital Clock : DigitalClock  SampleTime=Ts
  F_1 : Gain  Gain=F_1  Multiplication=Matrix(K*u) (u vector)
  F_2 : Gain  Gain=F_2  Multiplication=Matrix(K*u) (u vector)
  F_3 : Gain  Gain=F_3  Multiplication=Matrix(K*u) (u vector)
  F_4 : Gain  Gain=F_4  Multiplication=Matrix(K*u) (u vector)
  F_5 : Gain  Gain=F_5  Multiplication=Matrix(K*u) (u vector)
  F_6 : Gain  Gain=F_6  Multiplication=Matrix(K*u) (u vector)
  F_7 : Gain  Gain=F_7  Multiplication=Matrix(K*u) (u vector)
  F_8 : Gain  Gain=F_8  Multiplication=Matrix(K*u) (u vector)
  F_9 : Gain  Gain=F_9  Multiplication=Matrix(K*u) (u vector)
  Mpc : MATLAB Function  TreatAsAtomicUnit=on  SystemSampleTime=Ts
  Multiport Switch : MultiPortSwitch  Inputs=9
  Multiport Switch1 : MultiPortSwitch  Inputs=9
  Multiport Switch2 : MultiPortSwitch  Inputs=9
  Unit Delay : UnitDelay  InitialCondition=[0;0]  SampleTime=Ts
  U : Outport
  r(k+1) : Outport  Port=2
  Lambda : Outport  Port=3
  wires:
  Unit Delay/1 -> Mpc/1(U_delay)
  Constant1/1 -> Mpc/6(M)
  Mpc/1(U) -> U/1, Unit Delay/1
  Constant2/1 -> Mpc/7(Np)
  Rs/1 -> Mpc/12(Rs)
  Multiport Switch1/1 -> Mpc/5(Fxh)
  Multiport Switch2/1 -> Mpc/4(JF_part)
  Multiport Switch/1 -> Mpc/3(JE)
  Constant4/1 -> Mpc/8(U_min)
  Mpc/2(r) -> r(k+1)/1
  Digital Clock/1 -> Mpc/13(Tsim)
  Constant16/1 -> Mpc/9(U_max)
  Mpc/3(lambda) -> Lambda/1
  Velocity_updated/1 -> Mpc/11(Velocity_updated)
  Heading_updated/1 -> Mpc/10(Heading_updated)
  select_MPC/1 -> Multiport Switch1/1, Multiport Switch2/1, Mpc/2(select_MPC), Multiport Switch/1
  Constant12/1 -> Multiport Switch/2
  Constant17/1 -> Multiport Switch/3
  Constant22/1 -> Multiport Switch/4
  Constant9/1 -> Multiport Switch/5
  Constant10/1 -> Multiport Switch/6
  Constant6/1 -> Multiport Switch/7
  Constant18/1 -> Multiport Switch/8
  Constant7/1 -> Multiport Switch/9
  Constant20/1 -> Multiport Switch/10
  Constant23/1 -> Multiport Switch2/10
  Constant8/1 -> Multiport Switch2/9
  Constant21/1 -> Multiport Switch2/8
  Constant5/1 -> Multiport Switch2/7
  Constant13/1 -> Multiport Switch2/6
  Constant14/1 -> Multiport Switch2/5
  Constant3/1 -> Multiport Switch2/4
  Constant11/1 -> Multiport Switch2/3
  Constant19/1 -> Multiport Switch2/2
  F_7/1 -> Multiport Switch1/8
  F_3/1 -> Multiport Switch1/4
  F_6/1 -> Multiport Switch1/7
  F_5/1 -> Multiport Switch1/6
  F_9/1 -> Multiport Switch1/10
  F_1/1 -> Multiport Switch1/2
  F_2/1 -> Multiport Switch1/3
  F_4/1 -> Multiport Switch1/5
  F_8/1 -> Multiport Switch1/9
  Xh/1 -> F_5/1, F_4/1, F_3/1, F_2/1, F_1/1, F_9/1, F_8/1, F_7/1, F_6/1
  Constant15/1 -> Mpc/14(Tend)
  Constant26/1 -> Mpc/15(Ts)

== system ISReferenceApplication/Subsystem_1 ==
  select_MPC : Inport
  select_overlap : Inport  Port=2
  select_overlap2 : Inport  Port=3
  r(k+1) : Inport  Port=4
  Ui : Inport  Port=5
  i_pos : Inport  Port=6
  initial_Yi : Inport  Port=7
  Enable : EnablePort
  Mux : Mux  Inputs=2
  Subsystem : Subsystem
  Unit Delay1 : UnitDelay  InitialCondition=ro  SampleTime=Ts
  Unit Delay39 : UnitDelay  InitialCondition=ro  SampleTime=Ts
  gate1 : MATLAB Function  TreatAsAtomicUnit=on
  xhat : Outport
  Ysim : Outport  Port=2
  outputerror : Outport  Port=3
  systemerror : Outport  Port=4
  Ld : Outport  Port=5
  wires:
  Subsystem/2(Heading) -> Mux/2
  Subsystem/4(systemerror) -> systemerror/1
  Subsystem/5(Ld) -> Ld/1
  select_overlap/1 -> gate1/2(select_overlap)
  Subsystem/1("Velocity ") -> Mux/1
  r(k+1)/1 -> Unit Delay39/1
  Unit Delay39/1 -> Unit Delay1/1, Subsystem/3(r(k))
  Unit Delay1/1 -> Subsystem/4(r(k-1))
  select_MPC/1 -> gate1/1(select_MPC)
  gate1/1(state_MPC) -> Subsystem/1(select_MPC)
  select_overlap2/1 -> gate1/3(select_overlap2)
  Mux/1 -> Ysim/1
  gate1/2(state_overlap) -> Subsystem/2(select_overlap)
  Ui/1 -> Subsystem/5(U(k))
  Subsystem/6(xhat) -> xhat/1
  Subsystem/3(outputerror) -> outputerror/1
  initial_Yi/1 -> Subsystem/7(initial_Yi)
  i_pos/1 -> Subsystem/6(i_pos)

== system ISReferenceApplication/Subsystem_2 ==
  select_MPC : Inport
  select_overlap : Inport  Port=2
  select_overlap2 : Inport  Port=3
  r(k+1) : Inport  Port=4
  U : Inport  Port=5
  i_pos : Inport  Port=6
  initial_Yi : Inport  Port=7
  Enable : EnablePort
  Mux : Mux  Inputs=2
  Subsystem : Subsystem
  Unit Delay1 : UnitDelay  InitialCondition=ro  SampleTime=Ts
  Unit Delay39 : UnitDelay  InitialCondition=ro  SampleTime=Ts
  gate2 : MATLAB Function  TreatAsAtomicUnit=on
  xhat : Outport
  Y : Outport  Port=2
  outputerror : Outport  Port=3
  systemerror : Outport  Port=4
  Ld : Outport  Port=5
  wires:
  Mux/1 -> Y/1
  Subsystem/3(outputerror) -> outputerror/1
  Subsystem/4(systemerror) -> systemerror/1
  Subsystem/5(Ldt) -> Ld/1
  select_overlap/1 -> gate2/2(select_overlap)
  Subsystem/2(Handing) -> Mux/2
  r(k+1)/1 -> Unit Delay39/1
  Unit Delay39/1 -> Subsystem/3(r(k)), Unit Delay1/1
  Subsystem/6(xhat) -> xhat/1
  select_MPC/1 -> gate2/1(select_MPC)
  Subsystem/1(Velocity) -> Mux/1
  Unit Delay1/1 -> Subsystem/4(r(k-1))
  select_overlap2/1 -> gate2/3(select_overlap2)
  gate2/1(state_MPC) -> Subsystem/1(select_overlap)
  gate2/2(state_overlap) -> Subsystem/2(select_MPC)
  U/1 -> Subsystem/5(U(k))
  i_pos/1 -> Subsystem/6(i_pos)
  initial_Yi/1 -> Subsystem/7(initial_Yi)

== system ISReferenceApplication/Subsystem_3 ==
  select_MPC : Inport
  select_overlap : Inport  Port=2
  select_overlap2 : Inport  Port=3
  r(k+1) : Inport  Port=4
  U : Inport  Port=5
  i_pos : Inport  Port=6
  initial_Yi : Inport  Port=7
  Enable : EnablePort
  Mux : Mux  Inputs=2
  Subsystem : Subsystem
  Unit Delay1 : UnitDelay  InitialCondition=ro  SampleTime=Ts
  Unit Delay39 : UnitDelay  InitialCondition=ro  SampleTime=Ts
  gate3 : MATLAB Function  TreatAsAtomicUnit=on
  xhat : Outport
  Y : Outport  Port=2
  outputerror : Outport  Port=3
  systemerror : Outport  Port=4
  Ld : Outport  Port=5
  wires:
  Subsystem/4(systemerror) -> systemerror/1
  Subsystem/5(Ld) -> Ld/1
  select_overlap/1 -> gate3/2(select_overlap)
  Unit Delay1/1 -> Subsystem/4(r(k-1))
  Subsystem/2(Heading) -> Mux/2
  r(k+1)/1 -> Unit Delay39/1
  Unit Delay39/1 -> Unit Delay1/1, Subsystem/3(r(k))
  select_MPC/1 -> gate3/1(select_MPC)
  Subsystem/1(Velocity) -> Mux/1
  select_overlap2/1 -> gate3/3(select_overlap2)
  U/1 -> Subsystem/5(U(k))
  Mux/1 -> Y/1
  Subsystem/6(xhat) -> xhat/1
  Subsystem/3(outputerror) -> outputerror/1
  gate3/1(state_MPC) -> Subsystem/1(select_MPC)
  gate3/2(state_overlap) -> Subsystem/2(select_overlap)
  i_pos/1 -> Subsystem/6(i_pos)
  initial_Yi/1 -> Subsystem/7(initial_Yi)

== system ISReferenceApplication/Subsystem_4 ==
  select_MPC : Inport
  select_overlap : Inport  Port=2
  select_overlap2 : Inport  Port=3
  r(k+1) : Inport  Port=4
  U : Inport  Port=5
  i_pos : Inport  Port=6
  initial_Yi : Inport  Port=7
  Enable : EnablePort
  Mux : Mux  Inputs=2
  Subsystem : Subsystem
  Unit Delay1 : UnitDelay  InitialCondition=ro  SampleTime=Ts
  Unit Delay39 : UnitDelay  InitialCondition=ro  SampleTime=Ts
  gate4 : MATLAB Function  TreatAsAtomicUnit=on
  xhat : Outport
  Y : Outport  Port=2
  outputerror : Outport  Port=3
  systemerror : Outport  Port=4
  Ld : Outport  Port=5
  wires:
  Subsystem/4(systemerror) -> systemerror/1
  Subsystem/5(Ld) -> Ld/1
  Unit Delay1/1 -> Subsystem/4(r(k-1))
  Subsystem/2(Heading) -> Mux/2
  r(k+1)/1 -> Unit Delay39/1
  Unit Delay39/1 -> Unit Delay1/1, Subsystem/3(r(k))
  Subsystem/1(Velocity) -> Mux/1
  select_MPC/1 -> gate4/1(select_MPC)
  select_overlap/1 -> gate4/2(select_overlap)
  gate4/1(state_MPC) -> Subsystem/1(select_MPC)
  select_overlap2/1 -> gate4/3(select_overlap2)
  gate4/2(state_overlap) -> Subsystem/2(select_overlap)
  U/1 -> Subsystem/5(U(k))
  Mux/1 -> Y/1
  Subsystem/6(xhat) -> xhat/1
  Subsystem/3(outputerror) -> outputerror/1
  i_pos/1 -> Subsystem/6(i_pos)
  initial_Yi/1 -> Subsystem/7(initial_Yi)

== system ISReferenceApplication/Subsystem_5 ==
  select_MPC : Inport
  select_overlap : Inport  Port=2
  select_overlap2 : Inport  Port=3
  r(k+1) : Inport  Port=4
  U : Inport  Port=5
  i_pos : Inport  Port=6
  initial_Yi : Inport  Port=7
  Enable : EnablePort
  Mux : Mux  Inputs=2
  Subsystem : Subsystem
  Unit Delay1 : UnitDelay  InitialCondition=ro  SampleTime=Ts
  Unit Delay39 : UnitDelay  InitialCondition=ro  SampleTime=Ts
  gate5 : MATLAB Function  TreatAsAtomicUnit=on
  xhat : Outport
  Y : Outport  Port=2
  outputerror : Outport  Port=3
  systemerror : Outport  Port=4
  Ld : Outport  Port=5
  wires:
  Subsystem/4(systemerror) -> systemerror/1
  Subsystem/5(Ld) -> Ld/1
  select_overlap/1 -> gate5/2(select_overlap)
  Subsystem/2(Heading) -> Mux/2
  r(k+1)/1 -> Unit Delay39/1
  Subsystem/1(Velocity) -> Mux/1
  Unit Delay39/1 -> Unit Delay1/1, Subsystem/3(r(k))
  select_MPC/1 -> gate5/1(select_MPC)
  select_overlap2/1 -> gate5/3(select_overlap2)
  Unit Delay1/1 -> Subsystem/4(r(k-1))
  gate5/1(state_MPC) -> Subsystem/1(select_MPC)
  gate5/2(state_overlap) -> Subsystem/2(select_overlap)
  U/1 -> Subsystem/5(U(k))
  Mux/1 -> Y/1
  Subsystem/6(xhat) -> xhat/1
  Subsystem/3(outputerror) -> outputerror/1
  i_pos/1 -> Subsystem/6(i_pos)
  initial_Yi/1 -> Subsystem/7(initial_Yi)

== system ISReferenceApplication/Subsystem_6 ==
  select_MPC : Inport
  select_overlap : Inport  Port=2
  select_overlap2 : Inport  Port=3
  r(k+1) : Inport  Port=4
  U : Inport  Port=5
  i_pos : Inport  Port=6
  initial_Yi : Inport  Port=7
  Enable : EnablePort
  Mux : Mux  Inputs=2
  Subsystem : Subsystem
  Unit Delay1 : UnitDelay  InitialCondition=ro  SampleTime=Ts
  Unit Delay39 : UnitDelay  InitialCondition=ro  SampleTime=Ts
  gate6 : MATLAB Function  TreatAsAtomicUnit=on
  xhat : Outport
  Y : Outport  Port=2
  outputerror : Outport  Port=3
  systemerror : Outport  Port=4
  Ld : Outport  Port=5
  wires:
  Subsystem/4(systemerror) -> systemerror/1
  Subsystem/5(Ld) -> Ld/1
  gate6/1(state_MPC) -> Subsystem/1(select_MPC)
  select_overlap/1 -> gate6/2(select_overlap)
  Unit Delay1/1 -> Subsystem/4(r(k-1))
  Subsystem/2(Heading) -> Mux/2
  r(k+1)/1 -> Unit Delay39/1
  Unit Delay39/1 -> Unit Delay1/1, Subsystem/3(r(k))
  select_MPC/1 -> gate6/1(select_MPC)
  Subsystem/1(Velocity) -> Mux/1
  select_overlap2/1 -> gate6/3(select_overlap2)
  U/1 -> Subsystem/5(U(k))
  gate6/2(state_overlap) -> Subsystem/2(select_overlap)
  Mux/1 -> Y/1
  Subsystem/6(xhat) -> xhat/1
  Subsystem/3(outputerror) -> outputerror/1
  i_pos/1 -> Subsystem/6(i_pos)
  initial_Yi/1 -> Subsystem/7(initial_Yi)

== system ISReferenceApplication/Subsystem_7 ==
  select_MPC : Inport
  select_overlap : Inport  Port=2
  select_overlap2 : Inport  Port=3
  r(k+1) : Inport  Port=4
  U : Inport  Port=5
  i_pos : Inport  Port=6
  initial_Yi : Inport  Port=7
  Enable : EnablePort
  Mux : Mux  Inputs=2
  Subsystem : Subsystem
  Unit Delay1 : UnitDelay  InitialCondition=ro  SampleTime=Ts
  Unit Delay39 : UnitDelay  InitialCondition=ro  SampleTime=Ts
  gate7 : MATLAB Function  TreatAsAtomicUnit=on
  xhat : Outport
  Y : Outport  Port=2
  outputerror : Outport  Port=3
  systemerror : Outport  Port=4
  Ld : Outport  Port=5
  wires:
  Subsystem/4(systemerror) -> systemerror/1
  Subsystem/5(Ld) -> Ld/1
  gate7/1(state_MPC) -> Subsystem/1(select_MPC)
  select_overlap/1 -> gate7/2(select_overlap)
  Unit Delay1/1 -> Subsystem/4(r(k-1))
  Subsystem/2(Heading) -> Mux/2
  r(k+1)/1 -> Unit Delay39/1
  Unit Delay39/1 -> Unit Delay1/1, Subsystem/3(r(k))
  select_MPC/1 -> gate7/1(select_MPC)
  Subsystem/1(Velocity) -> Mux/1
  select_overlap2/1 -> gate7/3(select_overlap2)
  gate7/2(state_overlap) -> Subsystem/2(select_overlap)
  U/1 -> Subsystem/5(U(k))
  Mux/1 -> Y/1
  Subsystem/6(xhat) -> xhat/1
  Subsystem/3(outputerror) -> outputerror/1
  i_pos/1 -> Subsystem/6(i_pos)
  initial_Yi/1 -> Subsystem/7(initial_Yi)

== system ISReferenceApplication/Subsystem_8 ==
  select_MPC : Inport
  select_overlap : Inport  Port=2
  select_overlap2 : Inport  Port=3
  r(k+1) : Inport  Port=4
  U : Inport  Port=5
  i_pos : Inport  Port=6
  initial_Yi : Inport  Port=7
  Enable : EnablePort
  Mux : Mux  Inputs=2
  Subsystem : Subsystem
  Unit Delay1 : UnitDelay  InitialCondition=ro  SampleTime=Ts
  Unit Delay39 : UnitDelay  InitialCondition=ro  SampleTime=Ts
  gate8 : MATLAB Function  TreatAsAtomicUnit=on
  xhat : Outport
  Y : Outport  Port=2
  outputerror : Outport  Port=3
  systemerror : Outport  Port=4
  Ld : Outport  Port=5
  wires:
  Subsystem/4(systemerror) -> systemerror/1
  Subsystem/5(Ld) -> Ld/1
  gate8/1(state_MPC) -> Subsystem/1(select_MPC)
  select_overlap/1 -> gate8/2(select_overlap)
  Unit Delay1/1 -> Subsystem/4(r(k-1))
  Subsystem/2(Heading) -> Mux/2
  r(k+1)/1 -> Unit Delay39/1
  Unit Delay39/1 -> Unit Delay1/1, Subsystem/3(r(k))
  select_MPC/1 -> gate8/1(select_MPC)
  Subsystem/1(Velocity) -> Mux/1
  select_overlap2/1 -> gate8/3(select_overlap2)
  gate8/2(state_overlap) -> Subsystem/2(select_overlap)
  U/1 -> Subsystem/5(U(k))
  Mux/1 -> Y/1
  Subsystem/6(xhat) -> xhat/1
  Subsystem/3(outputerror) -> outputerror/1
  i_pos/1 -> Subsystem/6(i_pos)
  initial_Yi/1 -> Subsystem/7(initial_Yi)

== system ISReferenceApplication/Subsystem_9 ==
  select_MPC : Inport
  select_overlap : Inport  Port=2
  select_overlap2 : Inport  Port=3
  r(k+1) : Inport  Port=4
  U : Inport  Port=5
  i_pos : Inport  Port=6
  initial_Yi : Inport  Port=7
  Enable : EnablePort
  Mux : Mux  Inputs=2
  Subsystem : Subsystem
  Unit Delay1 : UnitDelay  InitialCondition=ro  SampleTime=Ts
  Unit Delay39 : UnitDelay  InitialCondition=ro  SampleTime=Ts
  gate9 : MATLAB Function  TreatAsAtomicUnit=on
  xhat : Outport
  Y : Outport  Port=2
  outputerror : Outport  Port=3
  systemerror : Outport  Port=4
  Ld : Outport  Port=5
  wires:
  Mux/1 -> Y/1
  Subsystem/3(outputerror) -> outputerror/1
  Subsystem/4(systemerror) -> systemerror/1
  Subsystem/5(Ld) -> Ld/1
  select_overlap/1 -> gate9/2(select_overlap)
  Unit Delay1/1 -> Subsystem/4(r(k-1))
  Subsystem/2(Heading) -> Mux/2
  r(k+1)/1 -> Unit Delay39/1
  Unit Delay39/1 -> Subsystem/3(r(k)), Unit Delay1/1
  Subsystem/6(xhat) -> xhat/1
  select_MPC/1 -> gate9/1(select_MPC)
  Subsystem/1(Velocity) -> Mux/1
  select_overlap2/1 -> gate9/3(select_overlap2)
  U/1 -> Subsystem/5(U(k))
  gate9/1(state_MPC) -> Subsystem/1(select_MPC)
  gate9/2(state_overlap) -> Subsystem/2(select_overlap)
  i_pos/1 -> Subsystem/6(i_pos)
  initial_Yi/1 -> Subsystem/7(initial_Yi)

== system ISReferenceApplication/VH2P ==
  Velocities : Inport
  HeadingAngles : Inport  Port=2
  Iintial Velocities : Inport  Port=3
  Iintial HeadingAngles : Inport  Port=4
  select_overlap : Inport  Port=5
  Initial position : Inport  Port=6
  Delay1 : Delay  DelayLength=1  InitialConditionSource=Input port  InitialCondition=0  ExternalReset=Rising  SampleTime=Ts
      settings: InputPortMap=u0,r5,p4
  Delay2 : Delay  DelayLength=1  InitialConditionSource=Input port  InitialCondition=0  ExternalReset=Rising  SampleTime=Ts
      settings: InputPortMap=u0,r5,p4
  Delay3 : Delay  DelayLength=1  InitialConditionSource=Input port  InitialCondition=0  ExternalReset=Rising  SampleTime=Ts
      settings: InputPortMap=u0,r5,p4
  From Workspace : FromWorkspace  VariableName=T_sim  SampleTime=Ts
  Unit Delay3 : UnitDelay  SampleTime=Ts
  YV2P : MATLAB Function  TreatAsAtomicUnit=on  SystemSampleTime=Ts
  Position : Outport
  wires:
  Velocities/1 -> YV2P/1(Velocity), Delay1/1
  HeadingAngles/1 -> Delay3/1, YV2P/3(Yaw)
  Delay2/1 -> YV2P/7(Lastpostion)
  Initial position/1 -> Delay2/3
  Iintial Velocities/1 -> Delay1/3
  Iintial HeadingAngles/1 -> Delay3/3
  From Workspace/1 -> YV2P/5(Tsim), Unit Delay3/1
  Delay1/1 -> YV2P/2(LastVelocity)
  Delay3/1 -> YV2P/4(LastYaw)
  Unit Delay3/1 -> YV2P/6(LastTsim)
  YV2P/1(Position) -> Delay2/1, Position/1
  select_overlap/1 -> Delay2/2, Delay1/2, Delay3/2

== system ISReferenceApplication/YV_update_Np1 ==
  XYplot_sim : Inport
  Velocity_sim : Inport  Port=2
  Heading_sim : Inport  Port=3
  From Workspace1 : FromWorkspace  VariableName=T_sim  SampleTime=Ts
  From Workspace3 : FromWorkspace  VariableName=XY_Ref_Upd  SampleTime=Ts
  MATLAB Function2 : MATLAB Function  TreatAsAtomicUnit=on  SystemSampleTime=Ts
  Velocity_updated : Outport
  Heading_updated : Outport  Port=2
  wires:
  MATLAB Function2/1(Velocity_updated) -> Velocity_updated/1
  From Workspace3/1 -> MATLAB Function2/1(XY_ref)
  MATLAB Function2/2(Heading_updated) -> Heading_updated/1
  From Workspace1/1 -> MATLAB Function2/5(Tsim)
  XYplot_sim/1 -> MATLAB Function2/2(XYplot_sim)
  Velocity_sim/1 -> MATLAB Function2/3(Velocity_sim)
  Heading_sim/1 -> MATLAB Function2/4(Yaw_sim)

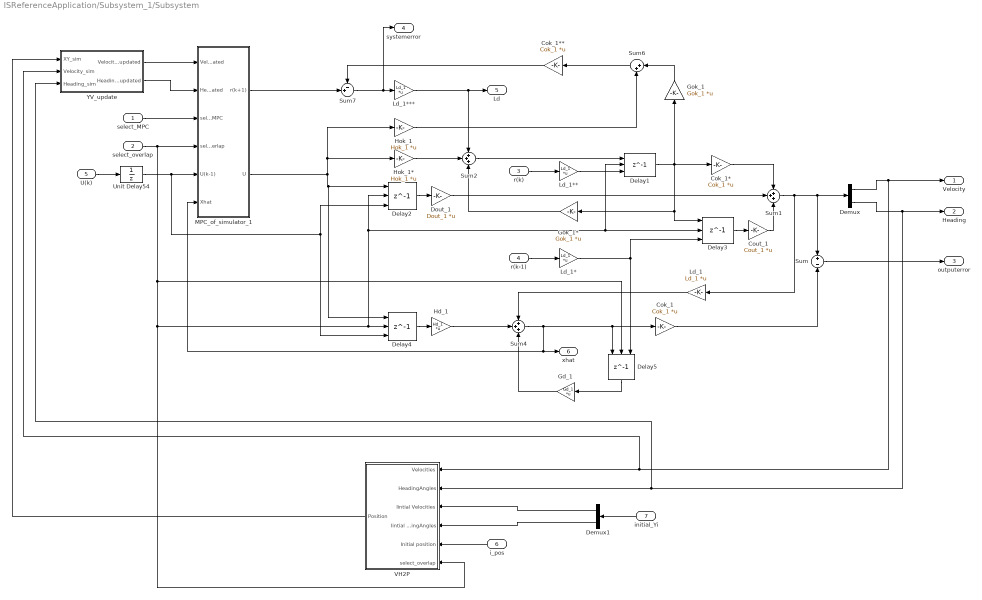
== system ISReferenceApplication/Subsystem_1/Subsystem ==
  select_MPC : Inport
  select_overlap : Inport  Port=2
  r(k) : Inport  Port=3
  r(k-1) : Inport  Port=4
  U(k) : Inport  Port=5
  i_pos : Inport  Port=6
  initial_Yi : Inport  Port=7
  Cok_1 : Gain  Gain=Cok_1  Multiplication=Matrix(K*u) (u vector)
  Cok_1* : Gain  Gain=Cok_1  Multiplication=Matrix(K*u) (u vector)
  Cok_1** : Gain  Gain=Cok_1  Multiplication=Matrix(K*u) (u vector)
  Cout_1 : Gain  Gain=Cout_1  Multiplication=Matrix(K*u) (u vector)
  Delay{1..5} (5 alike) : Delay  DelayLength=1  InitialConditionSource=Input port  InitialCondition=0  ExternalReset=Rising  SampleTime=Ts
      settings: InputPortMap=u0,r5,p4
  Demux : Demux  Outputs=2
  Demux1 : Demux  Outputs=2
  Dout_1 : Gain  Gain=Dout_1  Multiplication=Matrix(K*u) (u vector)
  Gd_1 : Gain  Gain=Gd_1  Multiplication=Matrix(K*u) (u vector)
  Gok_1 : Gain  Gain=Gok_1  Multiplication=Matrix(K*u) (u vector)
  Gok_1* : Gain  Gain=Gok_1  Multiplication=Matrix(K*u) (u vector)
  Hd_1 : Gain  Gain=Hd_1  Multiplication=Matrix(K*u) (u vector)
  Hok_1 : Gain  Gain=Hok_1  Multiplication=Matrix(K*u) (u vector)
  Hok_1* : Gain  Gain=Hok_1  Multiplication=Matrix(K*u) (u vector)
  Ld_1 : Gain  Gain=Ld_1  Multiplication=Matrix(K*u) (u vector)
  Ld_1* : Gain  Gain=Ld_1  Multiplication=Matrix(K*u) (u vector)
  Ld_1** : Gain  Gain=Ld_1  Multiplication=Matrix(K*u) (u vector)
  Ld_1*** : Gain  Gain=Ld_1  Multiplication=Matrix(K*u) (u vector)
  MPC_of_simulator_1 : Subsystem
  Sum : Sum  Inputs=+-
  Sum1 : Sum  Inputs=+++
  Sum2 : Sum  Inputs=+++
  Sum4 : Sum  Inputs=+++
  Sum6 : Sum  Inputs=|++
  Sum7 : Sum  Inputs=-+|
  Unit Delay54 : UnitDelay  SampleTime=Ts
  VH2P : Subsystem
  YV_update : Subsystem  TreatAsAtomicUnit=on
  "Velocity " : Outport
  Heading : Outport  Port=2
  outputerror : Outport  Port=3
  systemerror : Outport  Port=4
  Ld : Outport  Port=5
  xhat : Outport  Port=6
  wires:
  Gok_1*/1 -> Sum2/3
  Ld_1***/1 -> Ld/1, Sum2/1
  Cok_1**/1 -> Sum7/1
  Gok_1/1 -> Sum6/1
  r(k-1)/1 -> Ld_1*/1
  Sum7/1 -> Ld_1***/1, systemerror/1
  Sum6/1 -> Cok_1**/1
  Sum2/1 -> Delay1/1
  Delay3/1 -> Cout_1/1
  Delay2/1 -> Dout_1/1
  Cout_1/1 -> Sum1/3
  Delay1/1 -> Cok_1*/1, Delay3/1, Gok_1*/1, Gok_1/1
  Hok_1*/1 -> Sum2/2
  Dout_1/1 -> Sum1/2
  Ld_1**/1 -> Delay1/3
  Ld_1*/1 -> Delay3/3, Delay5/3
  Cok_1*/1 -> Sum1/1
  Hok_1/1 -> Sum6/2
  U(k)/1 -> Unit Delay54/1
  MPC_of_simulator_1/2(U) -> Hok_1/1, Hok_1*/1, Delay4/1, Delay2/1
  r(k)/1 -> Ld_1**/1
  Cok_1/1 -> Sum/2
  Delay5/1 -> Gd_1/1
  Gd_1/1 -> Sum4/3
  Delay4/1 -> Hd_1/1
  Hd_1/1 -> Sum4/2
  Sum1/1 -> Ld_1/1, Sum/1, Demux/1
  Sum4/1 -> Cok_1/1, Delay5/1, xhat/1, MPC_of_simulator_1/6(Xhat)
  Sum/1 -> outputerror/1
  MPC_of_simulator_1/1(r(k+1)) -> Sum7/2
  YV_update/1(Velocity_updated) -> MPC_of_simulator_1/1(Velocity_updated)
  YV_update/2(Heading_updated) -> MPC_of_simulator_1/2(Heading_updated)
  select_MPC/1 -> MPC_of_simulator_1/3(select_MPC)
  VH2P/1(Position) -> YV_update/1(XY_sim)
  Demux/2 -> YV_update/3(Heading_sim), VH2P/2(HeadingAngles), Heading/1
  Demux/1 -> YV_update/2(Velocity_sim), VH2P/1(Velocities), "Velocity "/1
  Unit Delay54/1 -> Delay4/3, Delay2/3, MPC_of_simulator_1/5(U(k-1))
  select_overlap/1 -> Delay5/2, VH2P/6(select_overlap), Delay1/2, Delay3/2, Delay2/2, Delay4/2, MPC_of_simulator_1/4(select_overlap)
  Ld_1/1 -> Sum4/1
  initial_Yi/1 -> Demux1/1
  i_pos/1 -> VH2P/5(Initial position)
  Demux1/1 -> VH2P/3(Iintial Velocities)
  Demux1/2 -> VH2P/4(Iintial HeadingAngles)

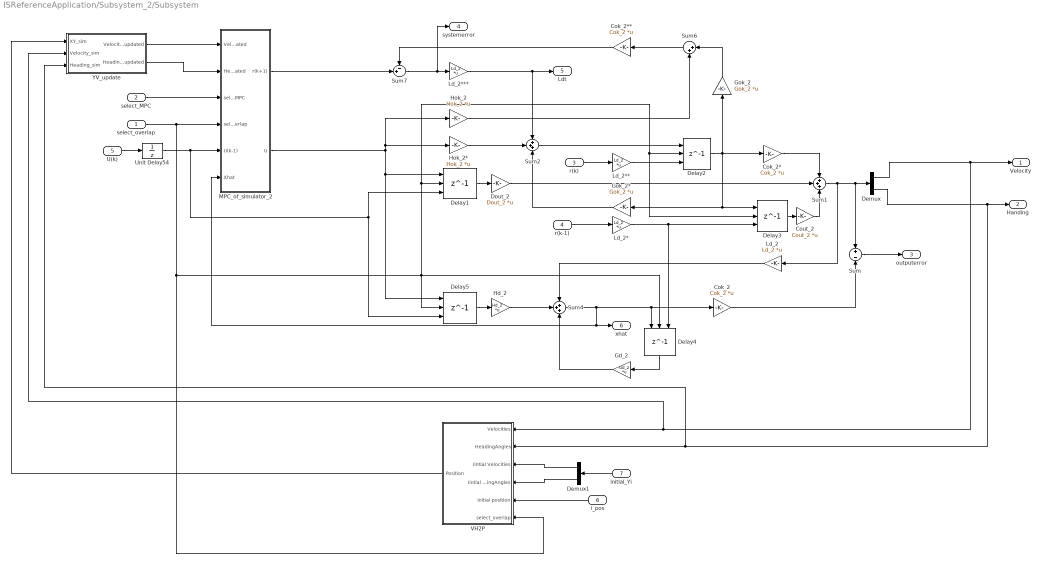
== system ISReferenceApplication/Subsystem_2/Subsystem ==
  select_overlap : Inport
  select_MPC : Inport  Port=2
  r(k) : Inport  Port=3
  r(k-1) : Inport  Port=4
  U(k) : Inport  Port=5
  i_pos : Inport  Port=6
  initial_Yi : Inport  Port=7
  Cok_2 : Gain  Gain=Cok_2  Multiplication=Matrix(K*u) (u vector)
  Cok_2* : Gain  Gain=Cok_2  Multiplication=Matrix(K*u) (u vector)
  Cok_2** : Gain  Gain=Cok_2  Multiplication=Matrix(K*u) (u vector)
  Cout_2 : Gain  Gain=Cout_2  Multiplication=Matrix(K*u) (u vector)
  Delay{1..5} (5 alike) : Delay  DelayLength=1  InitialConditionSource=Input port  InitialCondition=0  ExternalReset=Rising  SampleTime=Ts
      settings: InputPortMap=u0,r5,p4
  Demux : Demux  Outputs=2
  Demux1 : Demux  Outputs=2
  Dout_2 : Gain  Gain=Dout_2  Multiplication=Matrix(K*u) (u vector)
  Gd_2 : Gain  Gain=Gd_2  Multiplication=Matrix(K*u) (u vector)
  Gok_2 : Gain  Gain=Gok_2  Multiplication=Matrix(K*u) (u vector)
  Gok_2* : Gain  Gain=Gok_2  Multiplication=Matrix(K*u) (u vector)
  Hd_2 : Gain  Gain=Hd_2  Multiplication=Matrix(K*u) (u vector)
  Hok_2 : Gain  Gain=Hok_2  Multiplication=Matrix(K*u) (u vector)
  Hok_2* : Gain  Gain=Hok_2  Multiplication=Matrix(K*u) (u vector)
  Ld_2 : Gain  Gain=Ld_2  Multiplication=Matrix(K*u) (u vector)
  Ld_2* : Gain  Gain=Ld_2  Multiplication=Matrix(K*u) (u vector)
  Ld_2** : Gain  Gain=Ld_2  Multiplication=Matrix(K*u) (u vector)
  Ld_2*** : Gain  Gain=Ld_2  Multiplication=Matrix(K*u) (u vector)
  MPC_of_simulator_2 : Subsystem
  Sum : Sum  Inputs=+-
  Sum1 : Sum  Inputs=+++
  Sum2 : Sum  Inputs=+++
  Sum4 : Sum  Inputs=+++
  Sum6 : Sum  Inputs=|++
  Sum7 : Sum  Inputs=-+|
  Unit Delay54 : UnitDelay  SampleTime=Ts
  VH2P : Subsystem
  YV_update : Subsystem  TreatAsAtomicUnit=on
  Velocity : Outport
  Handing : Outport  Port=2
  outputerror : Outport  Port=3
  systemerror : Outport  Port=4
  Ldt : Outport  Port=5
  xhat : Outport  Port=6
  wires:
  Sum2/1 -> Delay2/1
  Cout_2/1 -> Sum1/3
  Dout_2/1 -> Sum1/2
  Sum6/1 -> Cok_2**/1
  Delay1/1 -> Dout_2/1
  MPC_of_simulator_2/2(U) -> Hok_2/1, Hok_2*/1, Delay1/1, Delay5/1
  Hok_2/1 -> Sum6/2
  Hok_2*/1 -> Sum2/2
  Gok_2*/1 -> Sum2/3
  r(k-1)/1 -> Ld_2*/1
  Gok_2/1 -> Sum6/1
  Cok_2**/1 -> Sum7/1
  select_overlap/1 -> MPC_of_simulator_2/4(select_overlap), VH2P/6(select_overlap), Delay4/2, Delay3/2, Delay2/2, Delay1/2, Delay5/2
  Delay3/1 -> Cout_2/1
  Ld_2*/1 -> Delay4/3, Delay3/3
  Sum7/1 -> Ld_2***/1, systemerror/1
  Delay2/1 -> Cok_2*/1, Delay3/1, Gok_2*/1, Gok_2/1
  Demux/1 -> YV_update/2(Velocity_sim), VH2P/1(Velocities), Velocity/1
  Cok_2*/1 -> Sum1/1
  Ld_2**/1 -> Delay2/3
  Unit Delay54/1 -> Delay1/3, Delay5/3, MPC_of_simulator_2/5(U(k-1))
  r(k)/1 -> Ld_2**/1
  Demux/2 -> YV_update/3(Heading_sim), VH2P/2(HeadingAngles), Handing/1
  Sum4/1 -> Delay4/1, Cok_2/1, MPC_of_simulator_2/6(Xhat), xhat/1
  Ld_2/1 -> Sum4/1
  Delay4/1 -> Gd_2/1
  Cok_2/1 -> Sum/2
  Delay5/1 -> Hd_2/1
  Gd_2/1 -> Sum4/3
  Hd_2/1 -> Sum4/2
  Ld_2***/1 -> Ldt/1, Sum2/1
  Sum1/1 -> Ld_2/1, Sum/1, Demux/1
  Sum/1 -> outputerror/1
  YV_update/1(Velocity_updated) -> MPC_of_simulator_2/1(Velocity_updated)
  YV_update/2(Heading_updated) -> MPC_of_simulator_2/2(Heading_updated)
  select_MPC/1 -> MPC_of_simulator_2/3(select_MPC)
  U(k)/1 -> Unit Delay54/1
  initial_Yi/1 -> Demux1/1
  VH2P/1(Position) -> YV_update/1(XY_sim)
  MPC_of_simulator_2/1(r(k+1)) -> Sum7/2
  i_pos/1 -> VH2P/5(Initial position)
  Demux1/1 -> VH2P/3(Iintial Velocities)
  Demux1/2 -> VH2P/4(Iintial HeadingAngles)

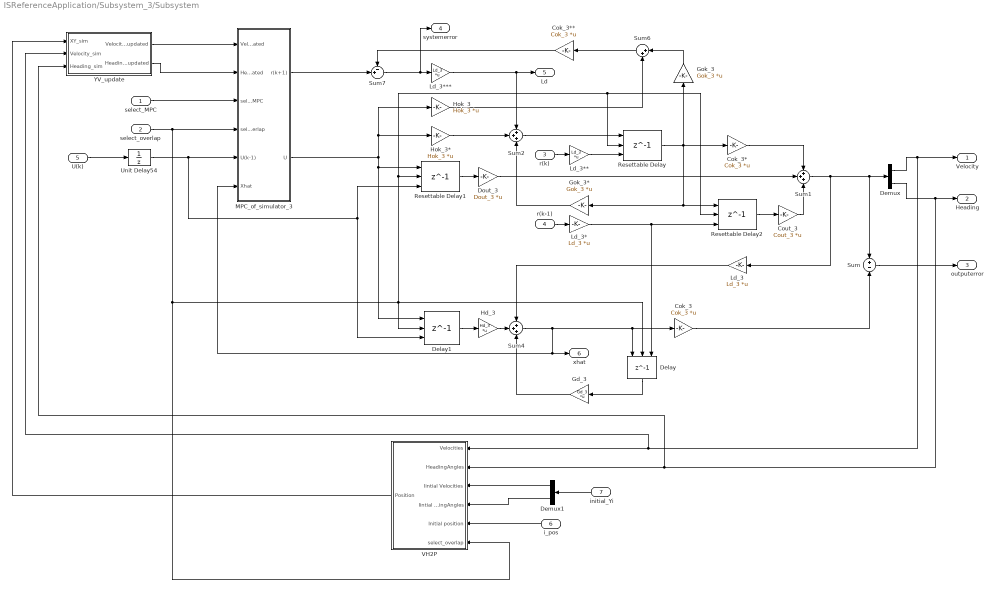
== system ISReferenceApplication/Subsystem_3/Subsystem ==
  select_MPC : Inport
  select_overlap : Inport  Port=2
  r(k) : Inport  Port=3
  r(k-1) : Inport  Port=4
  U(k) : Inport  Port=5
  i_pos : Inport  Port=6
  initial_Yi : Inport  Port=7
  Cok_3 : Gain  Gain=Cok_3  Multiplication=Matrix(K*u) (u vector)
  Cok_3* : Gain  Gain=Cok_3  Multiplication=Matrix(K*u) (u vector)
  Cok_3** : Gain  Gain=Cok_3  Multiplication=Matrix(K*u) (u vector)
  Cout_3 : Gain  Gain=Cout_3  Multiplication=Matrix(K*u) (u vector)
  Delay : Delay  DelayLength=1  InitialConditionSource=Input port  InitialCondition=0  ExternalReset=Rising  SampleTime=Ts
      settings: InputPortMap=u0,r5,p4
  Delay1 : Delay  DelayLength=1  InitialConditionSource=Input port  InitialCondition=0  ExternalReset=Rising  SampleTime=Ts
      settings: InputPortMap=u0,r5,p4
  Demux : Demux  Outputs=2
  Demux1 : Demux  Outputs=2
  Dout_3 : Gain  Gain=Dout_3  Multiplication=Matrix(K*u) (u vector)
  Gd_3 : Gain  Gain=Gd_3  Multiplication=Matrix(K*u) (u vector)
  Gok_3 : Gain  Gain=Gok_3  Multiplication=Matrix(K*u) (u vector)
  Gok_3* : Gain  Gain=Gok_3  Multiplication=Matrix(K*u) (u vector)
  Hd_3 : Gain  Gain=Hd_3  Multiplication=Matrix(K*u) (u vector)
  Hok_3 : Gain  Gain=Hok_3  Multiplication=Matrix(K*u) (u vector)
  Hok_3* : Gain  Gain=Hok_3  Multiplication=Matrix(K*u) (u vector)
  Ld_3 : Gain  Gain=Ld_3  Multiplication=Matrix(K*u) (u vector)
  Ld_3* : Gain  Gain=Ld_3  Multiplication=Matrix(K*u) (u vector)
  "Ld_3** " : Gain  Gain=Ld_3  Multiplication=Matrix(K*u) (u vector)
  Ld_3*** : Gain  Gain=Ld_3  Multiplication=Matrix(K*u) (u vector)
  MPC_of_simulator_3 : Subsystem
  Resettable Delay : Delay  DelayLength=1  InitialConditionSource=Input port  ExternalReset=Rising  SampleTime=Ts
      settings: InputPortMap=u0,r5,p4
  Resettable Delay1 : Delay  DelayLength=1  InitialConditionSource=Input port  ExternalReset=Rising  SampleTime=Ts
      settings: InputPortMap=u0,r5,p4
  Resettable Delay2 : Delay  DelayLength=1  InitialConditionSource=Input port  ExternalReset=Rising  SampleTime=Ts
      settings: InputPortMap=u0,r5,p4
  Sum : Sum  Inputs=+-
  Sum1 : Sum  Inputs=+++
  Sum2 : Sum  Inputs=+++
  Sum4 : Sum  Inputs=+++
  Sum6 : Sum  Inputs=|++
  Sum7 : Sum  Inputs=-+|
  Unit Delay54 : UnitDelay  SampleTime=Ts
  VH2P : Subsystem
  YV_update : Subsystem  TreatAsAtomicUnit=on
  Velocity : Outport
  Heading : Outport  Port=2
  outputerror : Outport  Port=3
  systemerror : Outport  Port=4
  Ld : Outport  Port=5
  xhat : Outport  Port=6
  wires:
  Sum2/1 -> Resettable Delay/1
  Resettable Delay1/1 -> Dout_3/1
  Dout_3/1 -> Sum1/2
  MPC_of_simulator_3/2(U) -> Hok_3/1, Hok_3*/1, Delay1/1, Resettable Delay1/1
  Cok_3**/1 -> Sum7/1
  Hok_3/1 -> Sum6/2
  Cout_3/1 -> Sum1/3
  r(k-1)/1 -> Ld_3*/1
  r(k)/1 -> "Ld_3** "/1
  Gok_3*/1 -> Sum2/3
  Sum7/1 -> Ld_3***/1, systemerror/1
  Cok_3*/1 -> Sum1/1
  Gok_3/1 -> Sum6/1
  "Ld_3** "/1 -> Resettable Delay/3
  U(k)/1 -> Unit Delay54/1
  Ld_3*/1 -> Resettable Delay2/3, Delay/3
  Resettable Delay2/1 -> Cout_3/1
  Hok_3*/1 -> Sum2/2
  Sum6/1 -> Cok_3**/1
  MPC_of_simulator_3/1(r(k+1)) -> Sum7/2
  Sum1/1 -> Ld_3/1, Sum/1, Demux/1
  Delay/1 -> Gd_3/1
  Gd_3/1 -> Sum4/3
  Cok_3/1 -> Sum/2
  Sum4/1 -> xhat/1, MPC_of_simulator_3/6(Xhat), Cok_3/1, Delay/1
  Hd_3/1 -> Sum4/2
  Delay1/1 -> Hd_3/1
  Ld_3***/1 -> Ld/1, Sum2/1
  Sum/1 -> outputerror/1
  Resettable Delay/1 -> Cok_3*/1, Resettable Delay2/1, Gok_3*/1, Gok_3/1
  YV_update/1(Velocity_updated) -> MPC_of_simulator_3/1(Velocity_updated)
  YV_update/2(Heading_updated) -> MPC_of_simulator_3/2(Heading_updated)
  select_overlap/1 -> MPC_of_simulator_3/4(select_overlap), Resettable Delay2/2, Resettable Delay/2, Resettable Delay1/2, Delay1/2, Delay/2, VH2P/6(select_overlap)
  VH2P/1(Position) -> YV_update/1(XY_sim)
  Demux/2 -> YV_update/3(Heading_sim), VH2P/2(HeadingAngles), Heading/1
  Demux/1 -> YV_update/2(Velocity_sim), VH2P/1(Velocities), Velocity/1
  select_MPC/1 -> MPC_of_simulator_3/3(select_MPC)
  Unit Delay54/1 -> Delay1/3, Resettable Delay1/3, MPC_of_simulator_3/5(U(k-1))
  Ld_3/1 -> Sum4/1
  initial_Yi/1 -> Demux1/1
  i_pos/1 -> VH2P/5(Initial position)
  Demux1/1 -> VH2P/3(Iintial Velocities)
  Demux1/2 -> VH2P/4(Iintial HeadingAngles)

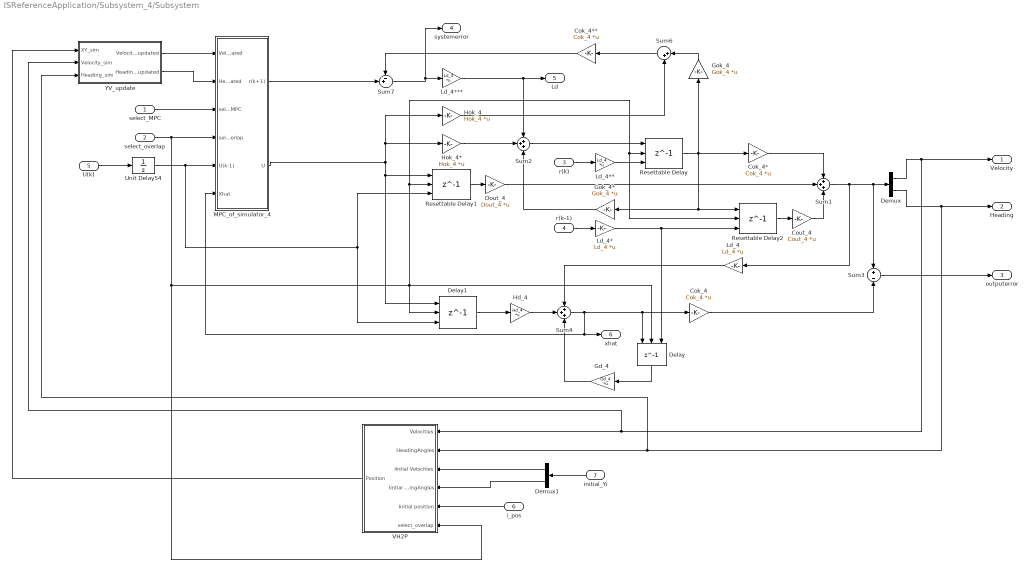
== system ISReferenceApplication/Subsystem_4/Subsystem ==
  select_MPC : Inport
  select_overlap : Inport  Port=2
  r(k) : Inport  Port=3
  r(k-1) : Inport  Port=4
  U(k) : Inport  Port=5
  i_pos : Inport  Port=6
  initial_Yi : Inport  Port=7
  Cok_4 : Gain  Gain=Cok_4  Multiplication=Matrix(K*u) (u vector)
  Cok_4* : Gain  Gain=Cok_4  Multiplication=Matrix(K*u) (u vector)
  Cok_4** : Gain  Gain=Cok_4  Multiplication=Matrix(K*u) (u vector)
  Cout_4 : Gain  Gain=Cout_4  Multiplication=Matrix(K*u) (u vector)
  Delay : Delay  DelayLength=1  InitialConditionSource=Input port  InitialCondition=0  ExternalReset=Rising  SampleTime=Ts
      settings: InputPortMap=u0,r5,p4
  Delay1 : Delay  DelayLength=1  InitialConditionSource=Input port  InitialCondition=0  ExternalReset=Rising  SampleTime=Ts
      settings: InputPortMap=u0,r5,p4
  Demux : Demux  Outputs=2
  Demux1 : Demux  Outputs=2
  Dout_4 : Gain  Gain=Dout_4  Multiplication=Matrix(K*u) (u vector)
  Gd_4 : Gain  Gain=Gd_4  Multiplication=Matrix(K*u) (u vector)
  Gok_4 : Gain  Gain=Gok_4  Multiplication=Matrix(K*u) (u vector)
  Gok_4* : Gain  Gain=Gok_4  Multiplication=Matrix(K*u) (u vector)
  Hd_4 : Gain  Gain=Hd_4  Multiplication=Matrix(K*u) (u vector)
  Hok_4 : Gain  Gain=Hok_4  Multiplication=Matrix(K*u) (u vector)
  Hok_4* : Gain  Gain=Hok_4  Multiplication=Matrix(K*u) (u vector)
  Ld_4 : Gain  Gain=Ld_4  Multiplication=Matrix(K*u) (u vector)
  Ld_4* : Gain  Gain=Ld_4  Multiplication=Matrix(K*u) (u vector)
  "Ld_4** " : Gain  Gain=Ld_4  Multiplication=Matrix(K*u) (u vector)
  Ld_4*** : Gain  Gain=Ld_4  Multiplication=Matrix(K*u) (u vector)
  MPC_of_simulator_4 : Subsystem
  Resettable Delay : Delay  DelayLength=1  InitialConditionSource=Input port  ExternalReset=Rising  SampleTime=Ts
      settings: InputPortMap=u0,r5,p4
  Resettable Delay1 : Delay  DelayLength=1  InitialConditionSource=Input port  ExternalReset=Rising  SampleTime=Ts
      settings: InputPortMap=u0,r5,p4
  Resettable Delay2 : Delay  DelayLength=1  InitialConditionSource=Input port  ExternalReset=Rising  SampleTime=Ts
      settings: InputPortMap=u0,r5,p4
  Sum1 : Sum  Inputs=+++
  Sum2 : Sum  Inputs=+++
  Sum3 : Sum  Inputs=+-
  Sum4 : Sum  Inputs=+++
  Sum6 : Sum  Inputs=|++
  Sum7 : Sum  Inputs=-+|
  Unit Delay54 : UnitDelay  SampleTime=Ts
  VH2P : Subsystem
  YV_update : Subsystem  TreatAsAtomicUnit=on
  Velocity : Outport
  Heading : Outport  Port=2
  outputerror : Outport  Port=3
  systemerror : Outport  Port=4
  Ld : Outport  Port=5
  xhat : Outport  Port=6
  wires:
  Ld_4*/1 -> Delay/3, Resettable Delay2/3
  Dout_4/1 -> Sum1/2
  Resettable Delay/1 -> Cok_4*/1, Resettable Delay2/1, Gok_4*/1, Gok_4/1
  Sum6/1 -> Cok_4**/1
  Sum7/1 -> systemerror/1, Ld_4***/1
  Gok_4/1 -> Sum6/1
  Cout_4/1 -> Sum1/3
  Gok_4*/1 -> Sum2/3
  Hok_4*/1 -> Sum2/2
  Hok_4/1 -> Sum6/2
  Resettable Delay2/1 -> Cout_4/1
  Sum2/1 -> Resettable Delay/1
  r(k)/1 -> "Ld_4** "/1
  Cok_4**/1 -> Sum7/1
  Ld_4***/1 -> Ld/1, Sum2/1
  Resettable Delay1/1 -> Dout_4/1
  r(k-1)/1 -> Ld_4*/1
  "Ld_4** "/1 -> Resettable Delay/3
  MPC_of_simulator_4/2(U) -> Hok_4/1, Hok_4*/1, Delay1/1, Resettable Delay1/1
  Cok_4*/1 -> Sum1/1
  Delay1/1 -> Hd_4/1
  Gd_4/1 -> Sum4/3
  Sum1/1 -> Ld_4/1, Sum3/1, Demux/1
  Sum4/1 -> Delay/1, Cok_4/1, MPC_of_simulator_4/6(Xhat), xhat/1
  Cok_4/1 -> Sum3/2
  Hd_4/1 -> Sum4/2
  Delay/1 -> Gd_4/1
  U(k)/1 -> Unit Delay54/1
  Sum3/1 -> outputerror/1
  select_MPC/1 -> MPC_of_simulator_4/3(select_MPC)
  MPC_of_simulator_4/1(r(k+1)) -> Sum7/2
  YV_update/1(Velocity_updated) -> MPC_of_simulator_4/1(Velocity_updated)
  YV_update/2(Heading_updated) -> MPC_of_simulator_4/2(Heading_updated)
  select_overlap/1 -> VH2P/6(select_overlap), Resettable Delay1/2, Resettable Delay2/2, Resettable Delay/2, Delay/2, Delay1/2, MPC_of_simulator_4/4(select_overlap)
  VH2P/1(Position) -> YV_update/1(XY_sim)
  Demux/2 -> YV_update/3(Heading_sim), VH2P/2(HeadingAngles), Heading/1
  Demux/1 -> VH2P/1(Velocities), YV_update/2(Velocity_sim), Velocity/1
  Unit Delay54/1 -> Resettable Delay1/3, Delay1/3, MPC_of_simulator_4/5(U(k-1))
  initial_Yi/1 -> Demux1/1
  Ld_4/1 -> Sum4/1
  i_pos/1 -> VH2P/5(Initial position)
  Demux1/1 -> VH2P/3(Iintial Velocities)
  Demux1/2 -> VH2P/4(Iintial HeadingAngles)
